simulink model "untitled"  (R2018b)
settings: Solver=VariableStepAuto  StartTime=0.0  StopTime=60  RelTol=1e-3
undefined symbols (not defined in the file or in its folder): K
libraries: simulink x1
settings Model: Creator=AlfredoMaussa  LastModifiedBy=AlfredoMaussa

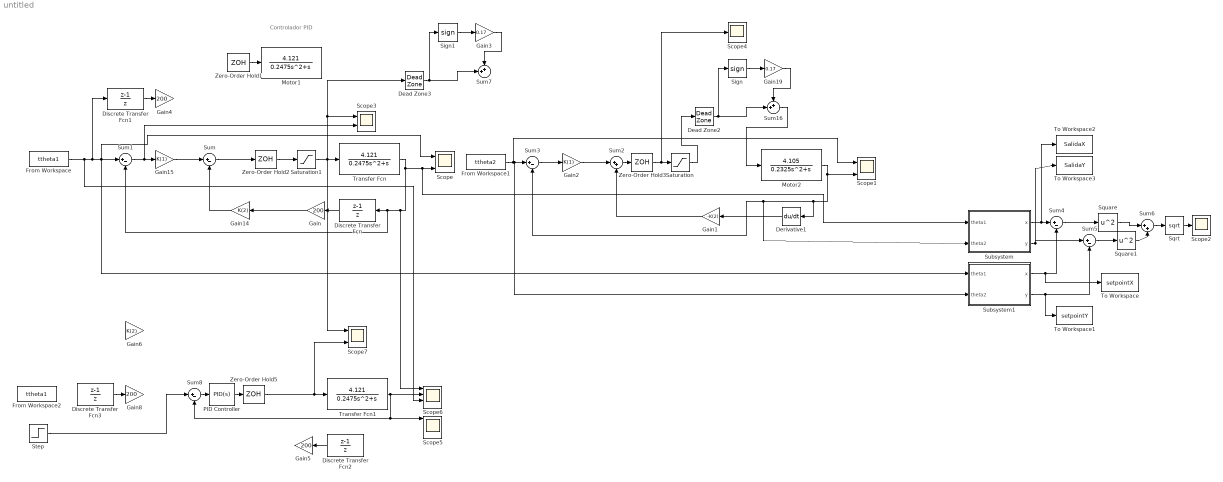
== system untitled ==
  note: Controlador PID
  Dead Zone2 : DeadZone  LowerValue=-0.17  UpperValue=0.17  SaturateOnIntegerOverflow=on
  Dead Zone3 : DeadZone  LowerValue=-0.17  UpperValue=0.17  SaturateOnIntegerOverflow=on
  Derivative1 : Derivative  CoefficientInTFapproximation=100
  Discrete Transfer Fcn{,1..3} (4 alike) : DiscreteTransferFcn  Numerator=[1,-1]  Denominator=[1 0]
  From Workspace : FromWorkspace  VariableName=ttheta1
  From Workspace1 : FromWorkspace  VariableName=ttheta2
  From Workspace2 : FromWorkspace  VariableName=ttheta1
  Gain{,4..5,8} (4 alike) : Gain  Gain=200
  Gain1 : Gain  Gain=-K(2)
  Gain14 : Gain  Gain=K(2)
  Gain15 : Gain  Gain=K(1)
  Gain19 : Gain  Gain=0.17
  Gain2 : Gain  Gain=K(1)
  Gain3 : Gain  Gain=0.17
  Gain6 : Gain  Gain=K(2)
  Motor1 : TransferFcn  Numerator=[4.121]  Denominator=[0.2475 1 0]
  Motor2 : TransferFcn  Numerator=[4.105]  Denominator=[0.2325 1 0]
  PID Controller : simulink/Continuous/PID Controller  Controller=PID  Form=Parallel  TimeDomain=Continuous-time  SampleTime=-1  IntegratorMethod=Forward Euler  FilterMethod=Forward Euler  ControllerParametersSource=internal  P=169.123999  I=1229.99272  D=6.48386314  UseFilter=on  N=100  TunerSelectOption=Transfer Function Based (PID Tuner App)  InitialConditionSource=internal  InitialConditionForIntegrator=0  InitialConditionForFilter=0  DifferentiatorICPrevScaledInput=0  ExternalReset=none  TrackingMode=off  Kt=1  LimitOutput=off  UpperSaturationLimit=inf  LowerSaturationLimit=-inf  LinearizeAsGain=on  AntiWindupMode=none  Kb=1  POutMin=[]  POutMax=[]  IOutMin=[]  IOutMax=[]  DOutMin=[]  DOutMax=[]  NOutMin=[]  NOutMax=[]  SumOutMin=[]  SumOutMax=[]  SaturationOutMin=[]  SaturationOutMax=[]  PParamMin=[]  PParamMax=[]  IParamMin=[]  IParamMax=[]  DParamMin=[]  DParamMax=[]  NParamMin=[]  NParamMax=[]  KbParamMin=[]  KbParamMax=[]  KtParamMin=[]  KtParamMax=[]  KbOutMin=[]  KbOutMax=[]  KtOutMin=[]  KtOutMax=[]  IntegratorOutMin=[]  IntegratorOutMax=[]  FilterOutMin=[]  FilterOutMax=[]  SumI1OutMin=[]  SumI1OutMax=[]  SumI2OutMin=[]  SumI2OutMax=[]  SumI3OutMin=[]  SumI3OutMax=[]  SumI4OutMin=[]  SumI4OutMax=[]  SumDOutMin=[]  SumDOutMax=[]  DifferentiatorOutMin=[]  DifferentiatorOutMax=[]  FilterDiffOutCoefMin=[]  FilterDiffOutCoefMax=[]  ReciprocalOutMin=[]  ReciprocalOutMax=[]  SumDenOutMin=[]  SumDenOutMax=[]  SumNumOutMin=[]  SumNumOutMax=[]  DivideOutMin=[]  DivideOutMax=[]  IntegratorContinuousStateAttributes=''  IntegratorStateMustResolveToSignalObject=off  IntegratorRTWStateStorageClass=Auto  FilterContinuousStateAttributes=''  FilterStateMustResolveToSignalObject=off  FilterRTWStateStorageClass=Auto  ParallelPVariant=InternalParameters  IdealPVariant=Disabled  IVariant=InternalParameters  DVariant=InternalParameters  IntegratorVariant=Continuous  SatVariant=Disabled  AWVariant=Passthrough  PCopyVariant=Disabled  TRVariant=Disabled  FdbkBlocksVariant=Forward  IdealPFdbkVariant=Disabled  SatFdbkVariant=Disabled  DerivativeFilterVariant=ContFilter  NVariant=InternalParameters  NCopyVariant=Disabled  FilterICVariant=InternalICsFilter  IntegratorICVariant=InternalICs  ExternalResetVariant=Disabled  TRSumVariant=Passthrough  SumFdbkVariant=Disabled  SumVariant=Sum_PID
  Saturation : Saturate  UpperLimit=1  LowerLimit=-1
  Saturation1 : Saturate  UpperLimit=1  LowerLimit=-1
  Scope{,1,3,7} (4 alike) : Scope  NumInputPorts=2
  Scope2 : Scope
  Scope4 : Scope
  Scope5 : Scope  NumInputPorts=4
  Scope6 : Scope  NumInputPorts=4
  Sign : Signum
  Sign1 : Signum
  Sqrt : Sqrt  SaturateOnIntegerOverflow=on
  Square : Math  Operator=square  SaturateOnIntegerOverflow=on
  Square1 : Math  Operator=square  SaturateOnIntegerOverflow=on
  Step : Step  SampleTime=0
  Subsystem : Subsystem
  Subsystem1 : Subsystem
  Sum{,1,3..5,8} (6 alike) : Sum  Inputs=|+-
  Sum16 : Sum  Inputs=++|
  Sum2 : Sum  Inputs=|++
  Sum6 : Sum  Inputs=|++
  Sum7 : Sum  Inputs=++|
  To Workspace : ToWorkspace  VariableName=setpointX  SampleTime=-1
  To Workspace1 : ToWorkspace  VariableName=setpointY  SampleTime=-1
  To Workspace2 : ToWorkspace  VariableName=SalidaX  SampleTime=-1
  To Workspace3 : ToWorkspace  VariableName=SalidaY  SampleTime=-1
  Transfer Fcn : TransferFcn  Numerator=[4.121]  Denominator=[0.2475 1 0]
  Transfer Fcn1 : TransferFcn  Numerator=[4.121]  Denominator=[0.2475 1 0]
  Zero-Order Hold{1..3,5} (4 alike) : ZeroOrderHold  SampleTime=0.005
  wires:
  Zero-Order Hold1/1 -> Motor1/1
  Transfer Fcn/1 -> Subsystem/1(theta1), Scope/2, Scope6/1, Discrete Transfer Fcn/1, Sum1/2
  Gain15/1 -> Sum/1
  Sum1/1 -> Scope3/2, Gain15/1
  Gain14/1 -> Sum/2
  Sum/1 -> Zero-Order Hold2/1
  Sum2/1 -> Zero-Order Hold3/1
  Gain1/1 -> Sum2/2
  Sum3/1 -> Gain2/1
  Gain2/1 -> Sum2/1
  Derivative1/1 -> Gain1/1
  From Workspace1/1 -> Scope1/1, Subsystem1/2(theta2), Sum3/1
  Motor2/1 -> Scope1/2, Subsystem/2(theta2), Sum3/2, Derivative1/1
  Subsystem/1(x) -> To Workspace2/1, Sum4/1
  Sum4/1 -> Square/1
  Sum5/1 -> Square1/1
  Subsystem/2(y) -> Sum5/1, To Workspace3/1
  Subsystem1/1(x) -> To Workspace/1, Sum4/2
  Subsystem1/2(y) -> To Workspace1/1, Sum5/2
  Square/1 -> Sum6/1
  Square1/1 -> Sum6/2
  Sum6/1 -> Sqrt/1
  Sqrt/1 -> Scope2/1
  Zero-Order Hold3/1 -> Scope4/1, Saturation/1
  Sum16/1 -> Motor2/1
  Dead Zone2/1 -> Sign/1, Sum16/2
  Sign/1 -> Gain19/1
  Gain19/1 -> Sum16/1
  Saturation/1 -> Dead Zone2/1
  Gain3/1 -> Sum7/1
  Sign1/1 -> Gain3/1
  Dead Zone3/1 -> Sum7/2, Sign1/1
  From Workspace/1 -> Scope6/3, Discrete Transfer Fcn1/1, Subsystem1/1(theta1), Sum1/1, Scope/1
  Discrete Transfer Fcn/1 -> Gain/1
  Gain/1 -> Gain14/1
  Saturation1/1 -> Scope7/1, Transfer Fcn/1, Scope3/1, Dead Zone3/1
  Discrete Transfer Fcn1/1 -> Gain4/1
  Discrete Transfer Fcn3/1 -> Gain8/1
  Discrete Transfer Fcn2/1 -> Gain5/1
  Transfer Fcn1/1 -> Scope5/1, Sum8/2, Scope6/2
  Sum8/1 -> PID Controller/1
  PID Controller/1 -> Zero-Order Hold5/1
  Zero-Order Hold2/1 -> Saturation1/1
  Zero-Order Hold5/1 -> Scope7/2, Transfer Fcn1/1
  Step/1 -> Sum8/1

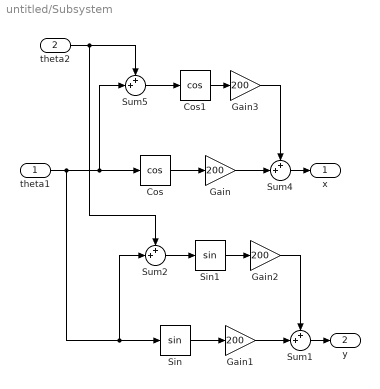
== system untitled/Subsystem ==
  theta1 : Inport
  theta2 : Inport  Port=2
  Cos : Trigonometry  Operator=cos
  Cos1 : Trigonometry  Operator=cos
  Gain{,1..3} (4 alike) : Gain  Gain=200
  Sin : Trigonometry
  Sin1 : Trigonometry
  Sum{1..2,4..5} (4 alike) : Sum  Inputs=++|
  x : Outport
  y : Outport  Port=2
  wires:
  Cos/1 -> Gain/1
  Sum4/1 -> x/1
  Gain3/1 -> Sum4/1
  Sum5/1 -> Cos1/1
  Gain/1 -> Sum4/2
  Cos1/1 -> Gain3/1
  Sin1/1 -> Gain2/1
  Gain1/1 -> Sum1/2
  theta2/1 -> Sum2/1, Sum5/1
  Sum2/1 -> Sin1/1
  Gain2/1 -> Sum1/1
  Sum1/1 -> y/1
  theta1/1 -> Sin/1, Sum2/2, Sum5/2, Cos/1
  Sin/1 -> Gain1/1

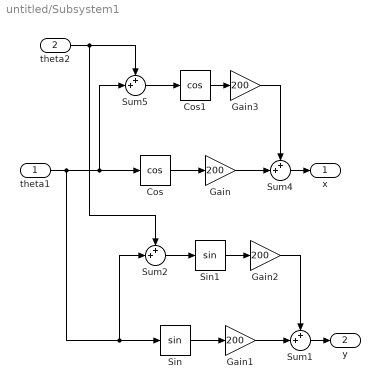
== system untitled/Subsystem1 ==
  theta1 : Inport
  theta2 : Inport  Port=2
  Cos : Trigonometry  Operator=cos
  Cos1 : Trigonometry  Operator=cos
  Gain{,1..3} (4 alike) : Gain  Gain=200
  Sin : Trigonometry
  Sin1 : Trigonometry
  Sum{1..2,4..5} (4 alike) : Sum  Inputs=++|
  x : Outport
  y : Outport  Port=2
  wires:
  Sin/1 -> Gain1/1
  theta1/1 -> Cos/1, Sum5/2, Sum2/2, Sin/1
  Sum1/1 -> y/1
  Gain2/1 -> Sum1/1
  Sum2/1 -> Sin1/1
  theta2/1 -> Sum5/1, Sum2/1
  Gain1/1 -> Sum1/2
  Sin1/1 -> Gain2/1
  Cos1/1 -> Gain3/1
  Gain/1 -> Sum4/2
  Sum5/1 -> Cos1/1
  Gain3/1 -> Sum4/1
  Sum4/1 -> x/1
  Cos/1 -> Gain/1
